simulink model "exp7"  (Simulink 8.1)
settings: Solver=ode45  StartTime=0.0  StopTime=5  RelTol=1e-3
libraries: powerlib x8, simulink x1
settings Model: Creator=sidharthbatchu  LastModifiedBy=sidharthbatchu
settings DataIOCC: SignalLoggingSaveFormat=Dataset
settings OptimizationCC: ExpressionDepthLimit=128
settings DebuggingCC: FcnCallInpInsideContextMsg=EnableAllAsError
settings GRTTargetCC: CombineOutputUpdateFcns=on  GRTInterface=off

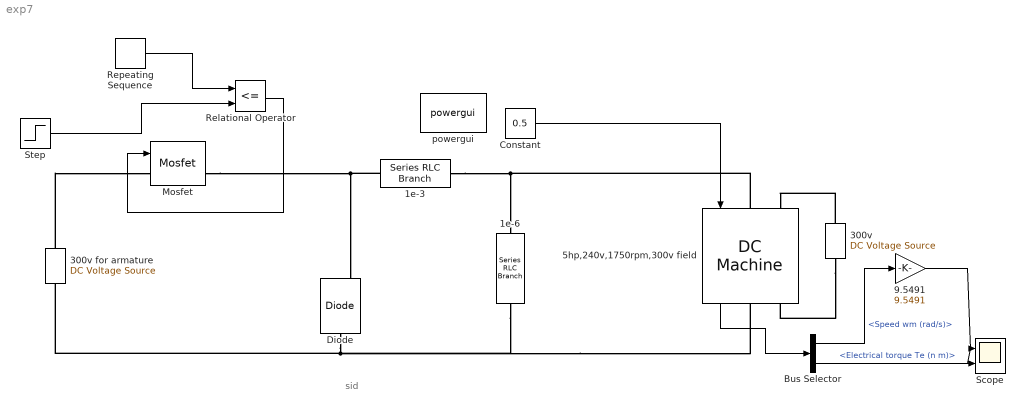
== system exp7 ==
  note: sid
  1e-3 : powerlib/Elements/Series RLC Branch  LConnTagsString=__new0  RConnTagsString=__new0  BranchType=L  Resistance=1  Inductance=1e-3  SetiL0=off  InitialCurrent=0  Capacitance=1e-6  Setx0=off  InitialVoltage=0  Measurements=None
  1e-6 : powerlib/Elements/Series RLC Branch  LConnTagsString=__new0  RConnTagsString=__new0  BranchType=C  Resistance=1  Inductance=1e-3  SetiL0=off  InitialCurrent=0  Capacitance=1e-6  Setx0=off  InitialVoltage=0  Measurements=None
  300v : powerlib/Electrical Sources/DC Voltage Source  Amplitude=300  Measurements=None
  "300v for armature " : powerlib/Electrical Sources/DC Voltage Source  Amplitude=300  Measurements=None
  5hp,240v,1750rpm,300v field : powerlib/Machines/DC Machine  PresetModel=01: 5HP 240V 1750RPM Field:300V  MechanicalLoad=Torque TL  FieldType=Wound  ShowDetailedParameters=on  RLa=[2.581 0.028]  RLf=[281.3 156]  Laf=0.9483  MachineConstant=Torque constant (N.m/A)  Ke=1.8  Kt=1.8  J=0.02215  Bm=0.002953  Tf=0.5161  w0=1  Ifinit=1  TsPowergui=0  TsBlock=-1
  9.5491 : Gain  Gain=9.5491
  Bus Selector : BusSelector  OutputSignals=Speed wm (rad/s),Electrical torque Te (n m)
  Constant : Constant  Value=0.5
  Diode : powerlib/Power Electronics/Diode  Ron=0.001  Lon=0  Vf=0.8  IC=0  UseSnubber=off  Rs=500  Cs=250e-9  Measurements=on
  Mosfet : powerlib/Power Electronics/Mosfet  Ron=0.1  Lon=0  Rd=0.01  Vfd=0  IC=0  Rs=1e5  Cs=inf  Measurements=on
  Relational Operator : RelationalOperator  Operator=<=  OutDataTypeStr=boolean
  Repeating Sequence : simulink/Sources/Repeating Sequence  rep_seq_t=[0 0.01e-3 0.02e-3]  rep_seq_y=[0 5 0]
  Scope : Scope  NumInputPorts=2
      settings: YMin=450~1  YMax=1100~10
  Step : Step  Time=02.5  Before=2  After=4  SampleTime=1
  powergui : powerlib/powergui  Priority=1  SimulationMode=Continuous  SolverType=Tustin  SampleTime=50e-6  frequency=60  SPID=off  DisableSnubberDevices=off  DisableRonSwitches=off  DisableVfSwitches=off  SwTol=0  Interpol=off  DisplayEquations=off  frequencyindice=0  Pbase=100e6  ErrMax=1e-4  Iterations=50  UnitsV=kV  UnitsW=MW  FunctionMessages=off  echomessages=off  HookPort=off  EnableUseOfTLC=off  x0status=blocks  RestoreLinks=warning  ResistiveCurrentMeasurement=off  Frange=[0:2:500]  Ylog=off  Xlog=on  ShowGrid=off  save=off  variable=ZData  ZoomFFT=off  StartTime=0.0  cycles=1  DisplayStyle=1  fundamental=60  FreqAxis=off  MaxFrequency=1000  frequencyindicesteady=1  RmsSteady=1  display=off  Ts=0  methode=off
  wires:
  Constant/1 -> 5hp,240v,1750rpm,300v field/1
  5hp,240v,1750rpm,300v field/1 -> Bus Selector/1
  Bus Selector/2 -> Scope/2  "<Electrical torque Te (n m)>"
  Bus Selector/1 -> 9.5491/1  "<Speed wm (rad/s)>"
  Repeating Sequence/1 -> Relational Operator/1
  Step/1 -> Relational Operator/2
  9.5491/1 -> Scope/1
  Relational Operator/1 -> Mosfet/1
  connections:
  "300v for armature "/RConn1 -- Mosfet/LConn1
  Mosfet/RConn1 -- 1e-3/LConn1 -- Diode/RConn1
  Diode/LConn1 -- 1e-6/RConn1 -- 5hp,240v,1750rpm,300v field/RConn1 -- "300v for armature "/LConn1
  1e-3/RConn1 -- 1e-6/LConn1 -- 5hp,240v,1750rpm,300v field/LConn1
  300v/RConn1 -- 5hp,240v,1750rpm,300v field/LConn2
  300v/LConn1 -- 5hp,240v,1750rpm,300v field/RConn2
